simulink subsystem "Model_propellers_forces"  (R2023a)
settings: Solver=VariableStepAuto  StartTime=0.0  StopTime=10.0  RelTol=1e-3
undefined symbols (not defined in the file): G_radu
settings Model: DefaultTestHarness=Model_propellers_forces_Harness  Creator=raduserseniuc  LastModifiedBy=raduserseniuc

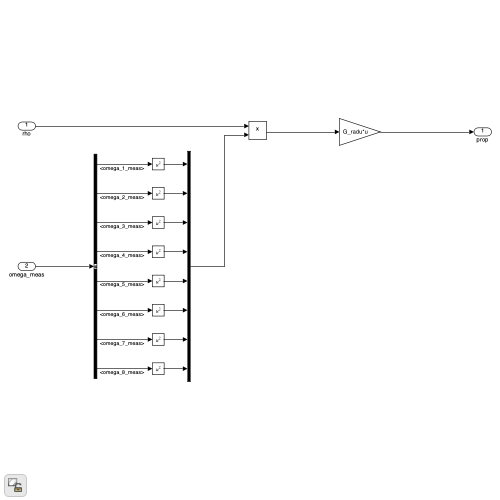
[thumbnail: Simulink's stored preview of the top-level diagram]
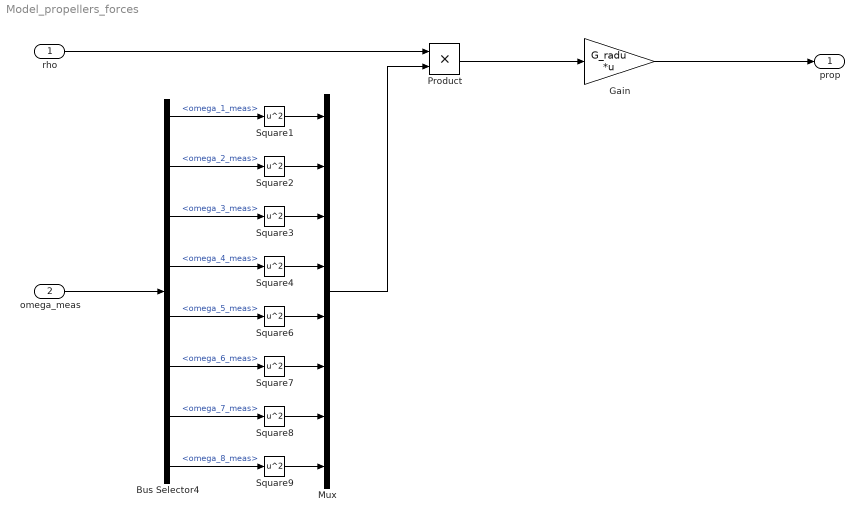
== system Model_propellers_forces ==
  rho : Inport
  omega_meas : Inport  Port=2
  Bus Selector4 : BusSelector  OutputSignals=omega_1_meas,omega_2_meas,omega_3_meas,omega_4_meas,omega_5_meas,omega_6_meas,omega_7_meas,omega_8_meas
  Gain : Gain  Gain=G_radu  Multiplication=Matrix(K*u)
  Mux : Mux  Inputs=8
  Product : Product
  Square{1..4,6..9} (8 alike) : Math  Operator=square
  prop : Outport
  wires:
  Gain/1 -> prop/1
  Product/1 -> Gain/1
  rho/1 -> Product/1
  Mux/1 -> Product/2
  Bus Selector4/8 -> Square9/1  "<omega_8_meas>"
  Bus Selector4/7 -> Square8/1  "<omega_7_meas>"
  Bus Selector4/6 -> Square7/1  "<omega_6_meas>"
  Bus Selector4/5 -> Square6/1  "<omega_5_meas>"
  Bus Selector4/4 -> Square4/1  "<omega_4_meas>"
  Bus Selector4/3 -> Square3/1  "<omega_3_meas>"
  Bus Selector4/2 -> Square2/1  "<omega_2_meas>"
  Bus Selector4/1 -> Square1/1  "<omega_1_meas>"
  Square4/1 -> Mux/4
  omega_meas/1 -> Bus Selector4/1
  Square7/1 -> Mux/6
  Square8/1 -> Mux/7
  Square9/1 -> Mux/8
  Square1/1 -> Mux/1
  Square3/1 -> Mux/3
  Square2/1 -> Mux/2
  Square6/1 -> Mux/5
